simulink model "sensor_flow_chart_failure"  (R2023b)
settings: Solver=VariableStepAuto  StartTime=0.0  StopTime=inf  RelTol=1e-3
settings Model: Creator=Beshary  LastModifiedBy=Beshary

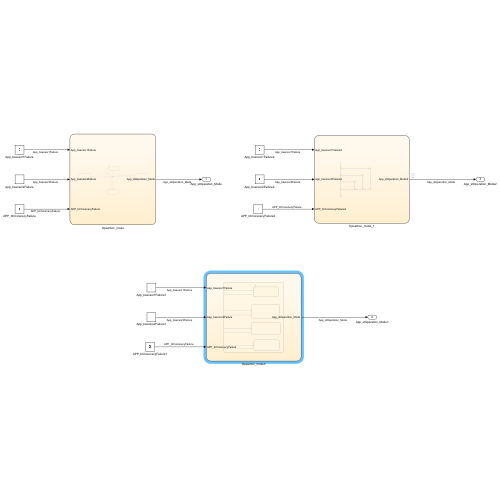
[thumbnail: Simulink's stored preview of the top-level diagram]
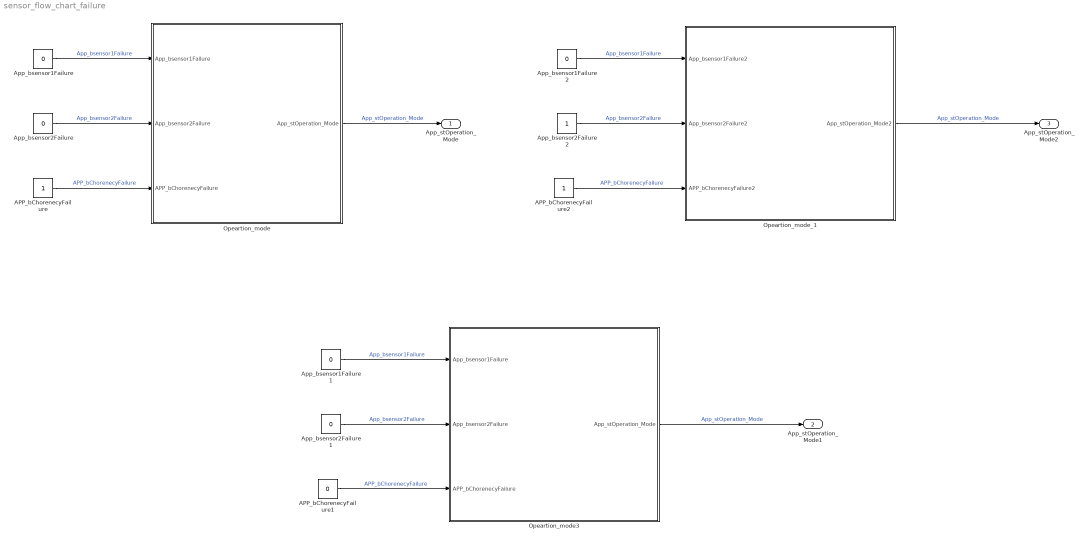
== system sensor_flow_chart_failure ==
  APP_bChorenecyFailure : Constant
  APP_bChorenecyFailure1 : Constant  Value=0
  APP_bChorenecyFailure2 : Constant
  App_bsensor1Failure : Constant  Value=0
  App_bsensor1Failure1 : Constant  Value=0
  App_bsensor1Failure2 : Constant  Value=0
  App_bsensor2Failure : Constant  Value=0
  App_bsensor2Failure1 : Constant  Value=0
  App_bsensor2Failure2 : Constant
  Opeartion_mode : Stateflow chart  TreatAsAtomicUnit=on
  Opeartion_mode3 : Stateflow chart  TreatAsAtomicUnit=on
  Opeartion_mode_1 : Stateflow chart  TreatAsAtomicUnit=on
  App_stOperation_Mode : Outport
  App_stOperation_Mode1 : Outport  Port=2
  App_stOperation_Mode2 : Outport  Port=3
  wires:
  App_bsensor1Failure/1 -> Opeartion_mode/1(App_bsensor1Failure)  "App_bsensor1Failure"
  App_bsensor2Failure/1 -> Opeartion_mode/2(App_bsensor2Failure)  "App_bsensor2Failure"
  APP_bChorenecyFailure/1 -> Opeartion_mode/3(APP_bChorenecyFailure)  "APP_bChorenecyFailure"
  Opeartion_mode/1(App_stOperation_Mode) -> App_stOperation_Mode/1  "App_stOperation_Mode"
  App_bsensor1Failure1/1 -> Opeartion_mode3/1(App_bsensor1Failure)  "App_bsensor1Failure"
  APP_bChorenecyFailure1/1 -> Opeartion_mode3/3(APP_bChorenecyFailure)  "APP_bChorenecyFailure"
  App_bsensor2Failure1/1 -> Opeartion_mode3/2(App_bsensor2Failure)  "App_bsensor2Failure"
  Opeartion_mode3/1(App_stOperation_Mode) -> App_stOperation_Mode1/1  "App_stOperation_Mode"
  Opeartion_mode_1/1(App_stOperation_Mode2) -> App_stOperation_Mode2/1  "App_stOperation_Mode"
  App_bsensor2Failure2/1 -> Opeartion_mode_1/2(App_bsensor2Failure2)  "App_bsensor2Failure"
  APP_bChorenecyFailure2/1 -> Opeartion_mode_1/3(APP_bChorenecyFailure2)  "APP_bChorenecyFailure"
  App_bsensor1Failure2/1 -> Opeartion_mode_1/1(App_bsensor1Failure2)  "App_bsensor1Failure"

== stateflow chart sensor_flow_chart_failure/Opeartion_mode ==
  state Normal
    en:
    App_stOperation_Mode=App_mode.Normal;
  state Downgraded_2
    en:
    App_stOperation_Mode=App_mode.DowngradedS2;
  state Downgraded_1
    en:
    App_stOperation_Mode=App_mode.DowngradedS1;
  state Failure
    en:
    App_stOperation_Mode=App_mode.Failure;
  (default) -> Normal
  Normal -> (junction 10) : [App_bsensor1Failure==1 ||App_bsensor2Failure==1||APP_bChorenecyFailure==1]
  (junction 10) -> Normal [order 1] : [App_bsensor1Failure==0 &&App_bsensor2Failure==0&&APP_bChorenecyFailure==0]
  Downgraded_1 -> (junction 10) : [App_bsensor1Failure==0 ||App_bsensor2Failure==1||APP_bChorenecyFailure==0]
  (junction 10) -> Downgraded_2 [order 4] : [App_bsensor1Failure==1 &&App_bsensor2Failure==0&&APP_bChorenecyFailure==1]
  (junction 10) -> Downgraded_1 [order 2] : [App_bsensor1Failure==0 &&App_bsensor2Failure==1&&APP_bChorenecyFailure==1]
  Downgraded_2 -> (junction 10) : [App_bsensor1Failure==1 ||App_bsensor2Failure==0||APP_bChorenecyFailure==0]
  Failure -> (junction 10) : [App_bsensor1Failure==0 ||App_bsensor2Failure==0||APP_bChorenecyFailure==0]
  (junction 10) -> Failure [order 3] : [App_bsensor1Failure==1 &&App_bsensor2Failure==1&&APP_bChorenecyFailure==1]
  data: App_bsensor1Failure input; App_bsensor2Failure input; APP_bChorenecyFailure input; App_stOperation_Mode output

== stateflow chart sensor_flow_chart_failure/Opeartion_mode3 ==
  state Modes
    state Normal
      en:
      App_stOperation_Mode=App_mode.Normal;
    state Downgraded_2
      en:
      App_stOperation_Mode=App_mode.DowngradedS2;
    state Downgraded_1
      en:
      App_stOperation_Mode=App_mode.DowngradedS1;
    state Failure
      en:
      App_stOperation_Mode=App_mode.Failure;
    (default) -> Normal
    Modes -> Normal [order 1] : [~APP_bChorenecyFailure]
    Normal -> Modes
    Modes -> Downgraded_2 [order 2] : [App_bsensor1Failure&&~App_bsensor1Failure]
    Downgraded_2 -> Modes
    Modes -> Downgraded_1 [order 3] : [~App_bsensor1Failure&&App_bsensor2Failure]
    Downgraded_1 -> Modes
    Modes -> Failure [order 4]
    Failure -> Modes
  data: App_bsensor1Failure input; App_bsensor2Failure input; APP_bChorenecyFailure input; App_stOperation_Mode output

== stateflow chart sensor_flow_chart_failure/Opeartion_mode_1 ==
  (default) -> (junction 35) : % Models_failure
  (junction 35) -> (junction 36) [order 1] : [APP_bChorenecyFailure2==0]
  (junction 35) -> (junction 37) [order 2]
  (junction 36) -> (junction 44) : {App_stOperation_Mode2=App_mode.Normal;}
  (junction 37) -> (junction 38) [order 1] : [App_bsensor2Failure2==1 &&App_bsensor1Failure2==0]
  (junction 37) -> (junction 39) [order 2]
  (junction 38) -> (junction 43) : {App_stOperation_Mode2=App_mode.DowngradedS2;}
  (junction 39) -> (junction 40) [order 1] : [App_bsensor1Failure2==0 &&App_bsensor2Failure2==1]
  (junction 39) -> (junction 41) [order 2] : {App_stOperation_Mode2=App_mode.Failure;}
  (junction 40) -> (junction 42) : {App_stOperation_Mode2=App_mode.DowngradedS1;}
  (junction 42) -> (junction 41)
  (junction 43) -> (junction 42)
  (junction 44) -> (junction 43)
  (junction 41) -> (junction 45)
  data: App_bsensor1Failure2 input; App_bsensor2Failure2 input; APP_bChorenecyFailure2 input; App_stOperation_Mode2 output
